simulink model "model"  (R2022a)
settings: Solver=ode4  StartTime=0.0  StopTime=100  FixedStep=0.01  RelTol=1e-3
undefined symbols (not defined in the file or in its folder): Serial_Port, Standard_Devices
libraries: sldrtlib x2, svdutilitieslib x2, nucleoutilitieslib x1
settings Model: SimulationMode=external  ExtModeTrigDuration=10000  Creator=Ali  LastModifiedBy=user
settings HardwareCC: ProdBitPerLong=64  ProdHWDeviceType=Intel->x86-64 (Linux 64)
settings ModelReferenceCC: EnableRefExpFcnMdlSchedulingChecks=off
settings RTWCC: Description=Simulink Desktop Real-Time  SystemTargetFile=sldrt.tlc  TemplateMakefile=sldrt.tmf  RTWCompilerOptimization=on
settings CodeAppCC: MaxIdLength=95
settings SimulinkDesktopRealTimeCC: TargetLibSuffix=_sldrt.a  TargetPreCompLibLocation=C:\Program Files\MATLAB\R2022a\toolbox\sldrt\lib\win64

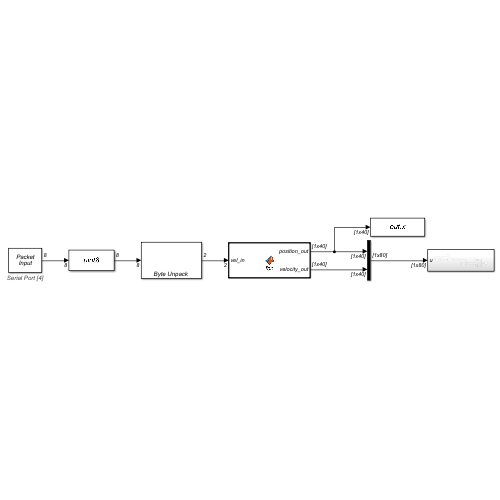
[thumbnail: Simulink's stored preview of the top-level diagram]
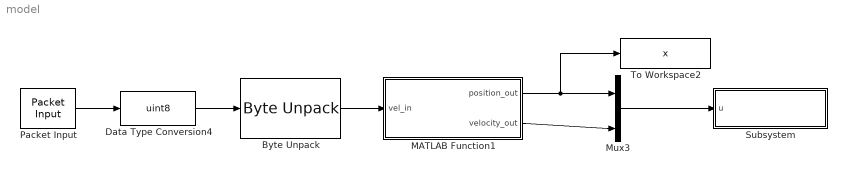
== system model ==
  Byte Unpack : nucleoutilitieslib/Byte Unpack  dimensions={[2]}  datatypes={'single'}  byteAlign=1  blockPlatform=nucleo
      settings: SourceProductBaseCode=ANDROID,ARDUINO,ML_ARDUINO,ECCORTEXA,ECCORTEXR,SC_BEAGLEBONE_BLUE,EC_FREEDOM_BOARD,EC_FRDM_K64F,INTEL_BLOCKSET,MICROBIT,NUCLEO,NVIDIA,PX4AUTOPILOTS,RASPPIIO,STMICRODIS,TIC2000,XILINX_BLOCKSET
  Data Type Conversion4 : DataTypeConversion  OutDataTypeStr=uint8  SaturateOnIntegerOverflow=off  RndMeth=Floor
  MATLAB Function1 : MATLAB Function  TreatAsAtomicUnit=on
  Mux3 : Mux  Inputs=2
  Packet Input : sldrtlib/Packet Input  SampleTime=0.01  MaxMissedTicks=10  ShowMissedTicks=off  YieldWhenWaiting=off  DrvName=Standard_Devices/Serial_Port  DrvAddress=4  DrvOptions=[115200 8 0 0 0 0 0 0]  PacketSize=8  DataTypes='8*uint8'  ShowReady=off  ShowError=off  PacketID=1  ByteOrder=1  ShowTimestamp=off
      settings: AttributesFormatString=Serial Port [4]
  Subsystem : Subsystem
  To Workspace2 : ToWorkspace  VariableName=x  SampleTime=-1
      settings: Save2DSignal=2-D array (concatenate along first dimension)
  wires:
  Packet Input/1 -> Data Type Conversion4/1
  Data Type Conversion4/1 -> Byte Unpack/1
  Byte Unpack/1 -> MATLAB Function1/1(vel_in)
  MATLAB Function1/1(position_out) -> To Workspace2/1, Mux3/1
  MATLAB Function1/2(velocity_out) -> Mux3/2
  Mux3/1 -> Subsystem/1(u)

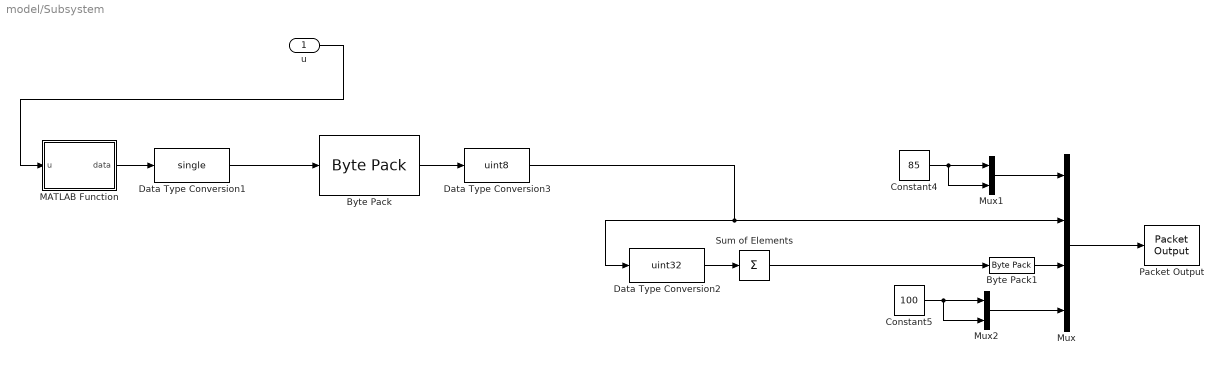
== system model/Subsystem ==
  u : Inport
  Byte Pack : svdutilitieslib/Byte Pack  maskPackedDataType=uint8  datatypes={'single'}  byteAlign=1  blockPlatform=arduinoert
      settings: SourceProductBaseCode=ANDROID,ARDUINO,ML_ARDUINO,ECCORTEXA,ECCORTEXR,SC_BEAGLEBONE_BLUE,EC_FREEDOM_BOARD,EC_FRDM_K64F,INTEL_BLOCKSET,MICROBIT,NUCLEO,NVIDIA,PX4AUTOPILOTS,RASPPIIO,STMICRODIS,TIC2000,XILINX_BLOCKSET
  Byte Pack1 : svdutilitieslib/Byte Pack  maskPackedDataType=uint8  datatypes={'uint32'}  byteAlign=1  blockPlatform=arduinoert
      settings: SourceProductBaseCode=ANDROID,ARDUINO,ML_ARDUINO,ECCORTEXA,ECCORTEXR,SC_BEAGLEBONE_BLUE,EC_FREEDOM_BOARD,EC_FRDM_K64F,INTEL_BLOCKSET,MICROBIT,NUCLEO,NVIDIA,PX4AUTOPILOTS,RASPPIIO,STMICRODIS,TIC2000,XILINX_BLOCKSET
  Constant4 : Constant  Value=85  OutDataTypeStr=uint8
  Constant5 : Constant  Value=100  OutDataTypeStr=uint8
  Data Type Conversion1 : DataTypeConversion  OutDataTypeStr=single  SaturateOnIntegerOverflow=off  RndMeth=Floor
  Data Type Conversion2 : DataTypeConversion  OutDataTypeStr=uint32  SaturateOnIntegerOverflow=off  RndMeth=Floor
  Data Type Conversion3 : DataTypeConversion  OutDataTypeStr=uint8  SaturateOnIntegerOverflow=off  RndMeth=Floor
  MATLAB Function : MATLAB Function  TreatAsAtomicUnit=on
  Mux : Mux
  Mux1 : Mux  Inputs=2
  Mux2 : Mux  Inputs=2
  Packet Output : sldrtlib/Packet Output  SampleTime=0.01  MaxMissedTicks=10  ShowMissedTicks=off  YieldWhenWaiting=off  DrvName=Standard_Devices/Serial_Port  DrvAddress=4  DrvOptions=[115200 8 0 0 0 0 0 0]  PacketSize=32  DataTypes='32*uint8'  ShowReady=off  ShowError=off  PacketID=1  ByteOrder=1  InitialValue=[]  FinalValue=[]
      settings: AttributesFormatString=Serial Port [4]
  Sum of Elements : Sum  Inputs=+
  wires:
  Constant4/1 -> Mux1/2, Mux1/1
  Constant5/1 -> Mux2/1, Mux2/2
  Data Type Conversion3/1 -> Mux/2, Data Type Conversion2/1
  Data Type Conversion1/1 -> Byte Pack/1
  Byte Pack1/1 -> Mux/3
  Data Type Conversion2/1 -> Sum of Elements/1
  Byte Pack/1 -> Data Type Conversion3/1
  Mux2/1 -> Mux/4
  Mux/1 -> Packet Output/1
  MATLAB Function/1(data) -> Data Type Conversion1/1
  Sum of Elements/1 -> Byte Pack1/1
  Mux1/1 -> Mux/1
  u/1 -> MATLAB Function/1(u)

== matlab function model/MATLAB Function1 ==
  data: position_out output; velocity_out output; vel_in input
function [position_out, velocity_out] = fcn(vel_in)

%%%%%%%% main Vasarhelyi Guidance Law %%%%%%%%

%% parameters %%
% x_arena: arena limits
x_arena = [-100, 100; ... % x wall
    -100, 100]; % y_wall
% spheres: obstacles
spheres = [0, 50, -50; 0, 10, 20; 5, 10, 2]; % x y radius
% agent_number: number of agents
agent_number = 20;
% Max radius of influence - Metric distance
radius = 20;
% time: simulation time

% dt: time step
dt = 0.01;


n = agent_number * 2;
persistent velocity position
if isempty(velocity)
    velocity = ones(1, n);
    position = randn(1, n)*20-10;
end


%% example of use of the function %%
%persistent position_array velocity_array
%if isempty(position_array)
%    position_array = zeros(2, n/2, time/dt);
%end
%if isempty(velocity_array)
%    velocity_array = zeros(2, n/2, time/dt);
%end

%for i = 1:time / dt
    r = radius;
    % Variables to be set
    is_active_migration = true;
    is_active_goal = false;
    is_active_arena = true;
    is_active_spheres = true;
    %is_active_cyl = false;
    circular = false;

    %%%%%%%%%%%%%%%%%%%%%%%%%%%%%%%%%%%%%%%%%%%%%%%%%%
    % Number of agents
    %
    %%%%%%%%%%%%%%%%%%%%%%%%%%%%%%%%%%%%%%%%%%%%%%%%%%
    %%%%%%%%%%%%%%%%%%%%%%%%%%%%%%%%%%%%%%%%%%%%%%%%%%
    % Max radius of influence - Metric distance
    %
    %%%%%%%%%%%%%%%%%%%%%%%%%%%%%%%%%%%%%%%%%%%%%%%%%%
    % add to input %

    %%%%%%%%%%%%%%%%%%%%%%%%%%%%%%%%%%%%%%%%%%%%%%%%%%
    % Max number of neighbors - Topological distance
    %
    %%%%%%%%%%%%%%%%%%%%%%%%%%%%%%%%%%%%%%%%%%%%%%%%%%


    %max_neig = 10;


    %%%%%%%%%%%%%%%%%%%%%%%%%%%%%%%%%%%%%%%%%%%%%%%%%%
    % Radius of collision -
    % it is the radius of the sphere that approximates
    % the drone. A collision is counted when two
    % spheres intersect.
    %%%%%%%%%%%%%%%%%%%%%%%%%%%%%%%%%%%%%%%%%%%%%%%%%%

    r_coll = 0.5;

    %%%%%%%%%%%%%%%%%%%%%%%%%%%%%%%%%%%%%%%%%%%%%%%%%%
    % Arena parameters - Cubic arena
    %
    %%%%%%%%%%%%%%%%%%%%%%%%%%%%%%%%%%%%%%%%%%%%%%%%%%

    % x,y,z positions of the walls
    % x_arena = [-100 100; % x wall
    %                    -100 100]; % y_wall
    %center_arena = sum(x_arena, 2) / 2;

    % Parameter that defines the influence radius of the arena repulsion force
    %d_arena = 1.5;

    % Constant of proportionality of the arena repulsion force
    %c_arena = .1;

    %%%%%%%%%%%%%%%%%%%%%%%%%%%%%%%%%%%%%%%%%%%%%%%%%%
    % Spheric obstacles parameters
    %
    %%%%%%%%%%%%%%%%%%%%%%%%%%%%%%%%%%%%%%%%%%%%%%%%%%

    % spheres = [0 10; 0 10; 5 10];

    n_spheres = length(spheres(1, :));

    %%%%%%%%%%%%%%%%%%%%%%%%%%%%%%%%%%%%%%%%%%%%%%%%%%
    % Reference values
    %
    %%%%%%%%%%%%%%%%%%%%%%%%%%%%%%%%%%%%%%%%%%%%%%%%%%

    % Inter-agent distance

    d_ref = 20;


    % Velocity direction
    u_ref = [1, 0, 0]';

    % Speed
    v_ref = 16;


    %%%%%%%%%%%%%%%%%%%%%%%%%%%%%%%%%%%%%%%%%%%%%%%%%%
    % Velocity and acceleration bounds for the agents
    %
    %%%%%%%%%%%%%%%%%%%%%%%%%%%%%%%%%%%%%%%%%%%%%%%%%%

    max_a = 10;
    max_v = 7;

    %%%%%%%%%%%%%%%%%%%%%%%%%%%%%%%%%%%%%%%%%%%%%%%%%%%%%%%%%%%%%%%%%%%%%%%%%%%
    % Vasarhelyi Paramteres
    %
    %%%%%%%%%%%%%%%%%%%%%%%%%%%%%%%%%%%%%%%%%%%%%%%%%%%%%%%%%%%%%%%%%%%%%%%%%%%

    %% Repulsion

    % Repulsion range
    r0_rep = d_ref; % radius of repulsion
    % Repulsion gain
    p_rep = 0.3;

    %% Friction

    % Stopping point offset of alignment
    r0_fric = 85.3;
    % Coefficient of velocity alignment
    C_fric = 0.05;
    % Velocity slack of alignement
    v_fric = 0.63;
    % Gain of braking curve
    p_fric = 3.2;
    % Acceleration of braking curve
    a_fric = 4.16;

    %% Obstacles and wall parameters

    % Stopping point offset of walls
    r0_shill = 0.1;
    % Velocity of virtual shill agents
    v_shill = 1.6;
    % Gain of bracking curve for walls
    p_shill = 0.55;
    % Acceleration of braking curve for walls
    a_shill = 3.02;
    r_agent = r_coll;
    % position: 1 x 2N vector of the positions of all the agents
    agent_number = floor(length(position)/2);
    agent_position = reshape(position, 2, agent_number);
    agent_velocity = reshape(velocity, 2, agent_number);
    pos = agent_position;
    vel = agent_velocity;

    % Initialize variables
    nb_agents = agent_number;
    M = zeros(nb_agents, nb_agents); % Neighborhood matrix
    dist_mat = zeros(nb_agents, nb_agents); % Distance matrix
    vel_rep = zeros(2, nb_agents); % Repulsion velocity
    vel_fric = zeros(2, nb_agents); % Velocity matching velocity
    vel_wall = zeros(2, nb_agents); % Arena repulsion velocity
    vel_obs = zeros(2, nb_agents); % Obstacle repulsion velocity
    vel_command = zeros(2, nb_agents); % Total commanded velocity

    nb_agent_collisions = 0; % Nb of collisions among agents
    nb_obs_collisions = 0; % Nb of collisions against obstacles
    min_dist_obs = 20;


    for agent = 1:nb_agents

        %% Find neighbors

        % Compute agent-agent distance matrix
        p_rel = pos - pos(:, agent);
        dist = sqrt(sum((p_rel.^2), 1));
        dist_mat(agent, :) = dist;

        % Define neighbours list
        neig_list = (1:nb_agents)';
        neig_list = neig_list(dist ~= 0);

        % Count collisions
        nb_agent_collisions = nb_agent_collisions + sum(dist < 2 * r_agent) - 1;

        % Initialize number of neighbours
        % nb_neig = nb_agents - 1;

        % Constraint on neighborhood given by the euclidean distance

        neig_list = neig_list(dist(neig_list) < r);
        nb_neig = length(neig_list);


        % Constraint on neighborhood given by the topological distance
        % if isfield(p_swarm, 'max_neig')
        %     if nb_neig > p_swarm.max_neig
        %         [~, idx] = sort(dist(neig_list));
        %         neig_list = neig_list(idx(1:p_swarm.max_neig));
        %         nb_neig = p_swarm.max_neig;
        %     end
        % end

        % Adjacency matrix (asymmetric in case of limited fov)
        M(agent, neig_list) = 1;

        %% Compute different contributions

        if nb_neig ~= 0
            v_rel = vel - vel(:, agent);
            v_rel_norm = sqrt(sum((v_rel.^2), 1));

            % Compute vel and pos unit vector between two agents
            p_rel_u = -p_rel ./ dist;
            v_rel_u = -v_rel ./ v_rel_norm;

            for agent2 =1:length(neig_list)

                % Repulsion and attraction
                if dist(neig_list(agent2)) < r0_rep % repulsion
                    vel_rep(:, agent) = vel_rep(:, agent) + ...
                        p_rep * (r0_rep - dist(neig_list(agent2))) * p_rel_u(:, neig_list(agent2));
                else % attraction
                    vel_rep(:, agent) = vel_rep(:, agent) + ...
                        p_rep * (dist(neig_list(agent2)) - r0_rep) * -p_rel_u(:, neig_list(agent2));
                end

                % Velocity alignement
                v_fric_max = get_v_max(v_fric, dist(neig_list(agent2))-r0_fric, a_fric, p_fric);

                if v_rel_norm(neig_list(agent2)) > v_fric_max
                    vel_fric(:, agent) = vel_fric(:, agent) + ...
                        C_fric * (v_rel_norm(neig_list(agent2)) - v_fric_max) * v_rel_u(:, neig_list(agent2));
                end
            end
        end

        %% Wall and obstacle avoidance

        % Add arena repulsion effect
        if (is_active_arena == true)
            unit = eye(2);
            %On each axis we have the two repulsions
            for axis = 1:2
                %On each axis there is two forces (each side of the arena)
                for dir = 1:2
                    dist_ab = abs(pos(axis, agent)-x_arena(axis, dir));

                    %Compute velocity of wall shill agent toward center of the arena
                    v_wall_virtual = unit(:, axis) .* v_shill;

                    if dir == 2
                        v_wall_virtual = -v_wall_virtual;
                    end

                    %Compute relative velocity (Wall - Agent)
                    vel_ab = sqrt(sum((vel(:, agent) - v_wall_virtual).^2));

                    v_wall_max = get_v_max(0, dist_ab-r0_shill, a_shill, p_shill);

                    if vel_ab > v_wall_max
                        vel_wall(:, agent) = vel_wall(:, agent) + ...
                            (vel_ab - v_wall_max) * (v_wall_virtual - vel(:, agent)) ./ vel_ab;
                    end
                end
            end
        end

        % Compute spheric effect
        if (is_active_spheres == true)

            for obs = 1:n_spheres
                % Get obstacle center and radius
                c_obs = spheres(1:2, obs);
                r_obs = spheres(3, obs);

                % Compute distance agent(a)-obstacle(b)
                dist_ab = sqrt(sum((pos(:, agent) - c_obs).^2)) - r_obs;
                nb_obs_collisions = nb_obs_collisions + sum(dist_ab < r_agent);

                % Set the virtual speed of the obstacle direction out of
                % the obstacle
                v_obs_virtual = (pos(:, agent) - c_obs) / (dist_ab + r_obs) * v_shill;

                % Compute relative velocity agent-obstacle
                vel_ab = sqrt(sum((vel(:, agent) - v_obs_virtual).^2));

                if dist_ab < min_dist_obs
                    min_dist_obs = dist_ab;
                end

                v_obs_max = get_v_max(0, dist_ab-r0_shill, a_shill, p_shill);

                if vel_ab > v_obs_max
                    vel_obs(:, agent) = vel_obs(:, agent) + (vel_ab - v_obs_max) * (v_obs_virtual - vel(:, agent)) ./ vel_ab;
                end
            end
        end

        %% Sum agent-agent and obstacle contributions

        vel_command(:, agent) = vel_rep(:, agent) + vel_fric(:, agent) + vel_obs(:, agent) + vel_wall(:, agent);

        % Add self propulsion OR migration term
        v_norm = sqrt(sum((vel(:, agent).^2), 1));

        if is_active_migration == false % migration
            vel_command(:, agent) = vel_command(:, agent) + v_ref * u_ref;
        elseif is_active_goal == true
            x_goal_rel = x_goal - pos(:, agent);
            u_goal = x_goal_rel / norm(x_goal_rel);
            vel_command(:, agent) = vel_command(:, agent) + v_ref * u_goal;
        else
            % self-propulsion
            if v_norm > 0
                vel_command(:, agent) = vel_command(:, agent) + v_ref * vel(:, agent) / v_norm;
            end
        end
    end

    %% random effect
    vel_command = vel_command + 0 * randn(2, nb_agents);

    %% bound velocities and accelerations

    % Bound velocities and acceleration
    if ~isempty(max_v)
        vel_cmd_norm = sqrt(sum((vel_command.^2), 1));
        % v_norm = sqrt(sum((vel.^2), 1));

        idx_to_bound = (vel_cmd_norm > max_v);
        if sum(idx_to_bound) > 0
            vel_command(:, idx_to_bound) = max_v * ...
                vel_command(:, idx_to_bound) ./ repmat(vel_cmd_norm(idx_to_bound), 2, 1);
        end
    end
    %if ~isempty(max_a)
    %    accel_cmd = (vel_command - vel) ./ dt;
    %    accel_cmd_norm = sqrt(sum(accel_cmd.^2, 1));
    %    idx_to_bound = (accel_cmd_norm > max_a | accel_cmd_norm < -max_a);
    %    if sum(idx_to_bound) > 0
    %        vel_command(:, idx_to_bound) = vel(:, idx_to_bound) + ...
    %            dt * max_a * accel_cmd(:, idx_to_bound) ./ ...
    %            repmat(accel_cmd_norm(idx_to_bound), 2, 1);
    %    end
    %end

    % add velocity to each agent to move circularly
    if circular
        % v_circular = 0.5;
        angle = atan2(pos(2, :), pos(1, :));
        vel_command = vel_command + repmat(v_circular, 2, 1) .* [-sin(angle); cos(angle)];
    end

    % vel_command = vel_command +
    velocity_law = reshape(vel_command, 1, 2*nb_agents);

    velocity_out = velocity_law;
    v_command = velocity_law;
    v_command(1:2) = vel_in;

    position = position + v_command * dt;
    position_out = position;
    %position_array(:, :, i) = reshape(position, 2, n/2);
    %velocity_array(:, :, i) = reshape(v_command, 2, n/2);
    velocity = v_command;
%end
% plot_results(agent_number, position_array, x_arena, spheres);
% step_time = 1;
% graph_animation_creator(agent_number, position_array, x_arena, spheres,...
%     step_time, dt, radius);
%plot_results_timeline(agent_number, position_array, velocity_array, ...
%    x_arena, spheres);






y = position;
end

%%%%%%%%%%%%%%%%%%%%%%%%%%%%%%%%%%%%%%%%%%%%%%%%%
% Calculate V fric max
%
%%%%%%%%%%%%%%%%%%%%%%%%%%%%%%%%%%%%%%%%%%%%%%%%%

function [v_fricmax] = get_v_max(v_fric, r, a, p)

if r < 0
    v_fricmax = 0;
elseif r * p > 0 && r * p < a / p
    v_fricmax = r * p;
else
    v_fricmax = sqrt(2*a*r-a^2/p^2);
end

if v_fricmax < v_fric
    v_fricmax = v_fric;
end
end

== matlab function model/Subsystem/MATLAB Function ==
  data: u input; data output
function data = fcn(u)
persistent iteration
if isempty(iteration)
    iteration = 0;
end
data = zeros(1, 6);
for i = 1:6
    iteration = iteration + 1;
    data(i) = u(iteration);
    if iteration >= length(u)
        iteration = 0;
    end
end
